simulink model "electromech_dynamics"  (R2020b)
settings: Solver=VariableStepAuto  StartTime=0.0  StopTime=10.0  RelTol=1e-3
values from neighbouring files (symbols this model uses):
  ms22g = 1/g    (= 0.101936799185)    [balrob_params.m]
  Ts = 1e-2    (= 0.01)    [balrob_params.m]
undefined symbols (not defined in the file or in its folder): C12qq_coeff, drv, Fv1, g2_coeff, gbox, M11q, M12q_coeff, M22q, sens, ua2tau1
settings Model: Creator=gioel  LastModifiedBy=gioel

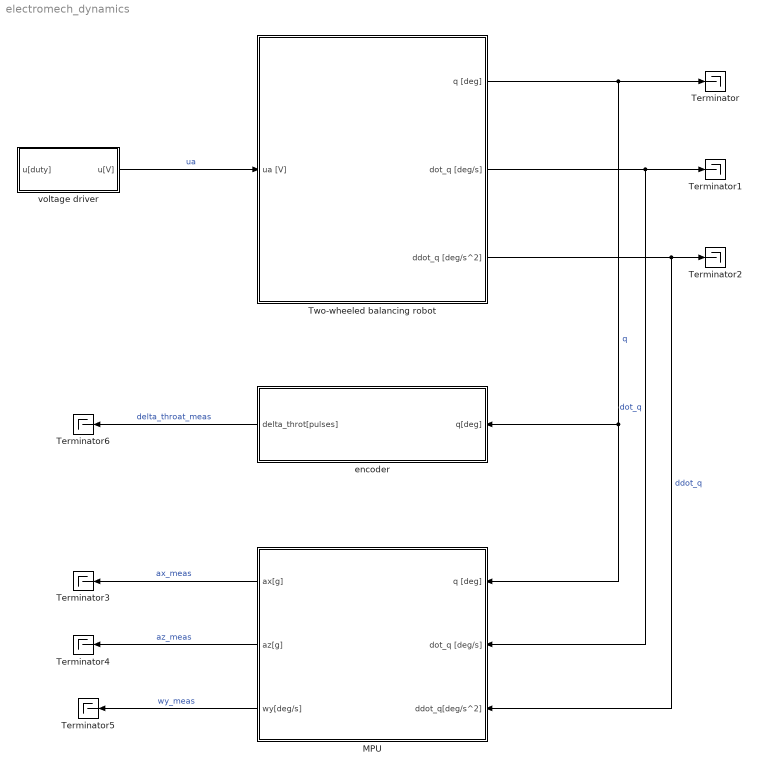
== system electromech_dynamics ==
  MPU : Subsystem
  Terminator{,1..6} (7 alike) : Terminator
  Two-wheeled balancing robot : Subsystem
  encoder : Subsystem
  voltage driver : Subsystem
  wires:
  voltage driver/1(u[V]) -> Two-wheeled balancing robot/1(ua [V])  "ua"
  Two-wheeled balancing robot/1(q [deg]) -> MPU/1(q [deg]), encoder/1(q[deg]), Terminator/1  "q"
  Two-wheeled balancing robot/3(ddot_q [deg/s^2]) -> MPU/3(ddot_q[deg/s^2]), Terminator2/1  "ddot_q"
  Two-wheeled balancing robot/2(dot_q [deg/s]) -> MPU/2(dot_q [deg/s]), Terminator1/1  "dot_q"
  MPU/1(ax[g]) -> Terminator3/1  "ax_meas"
  encoder/1(delta_throt[pulses]) -> Terminator6/1  "delta_throat_meas"
  MPU/2(az[g]) -> Terminator4/1  "az_meas"
  MPU/3(wy[deg/s]) -> Terminator5/1  "wy_meas"

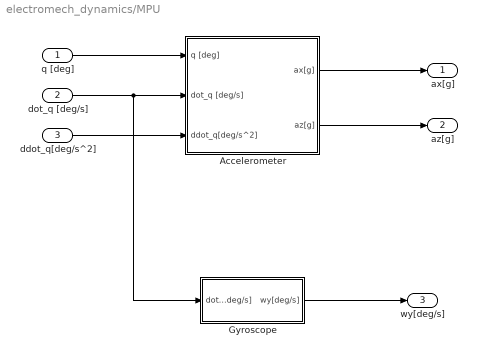
== system electromech_dynamics/MPU ==
  q [deg] : Inport
  dot_q [deg/s] : Inport  Port=2
  ddot_q[deg/s^2] : Inport  Port=3
  Accelerometer : Subsystem
  Gyroscope : Subsystem
  ax[g] : Outport
  az[g] : Outport  Port=2
  wy[deg/s] : Outport  Port=3
  wires:
  q [deg]/1 -> Accelerometer/1(q [deg])
  dot_q [deg/s]/1 -> Gyroscope/1(dot_q [deg/s]), Accelerometer/2(dot_q [deg/s])
  ddot_q[deg/s^2]/1 -> Accelerometer/3(ddot_q[deg/s^2])
  Gyroscope/1(wy[deg/s]) -> wy[deg/s]/1
  Accelerometer/1(ax[g]) -> ax[g]/1
  Accelerometer/2(az[g]) -> az[g]/1

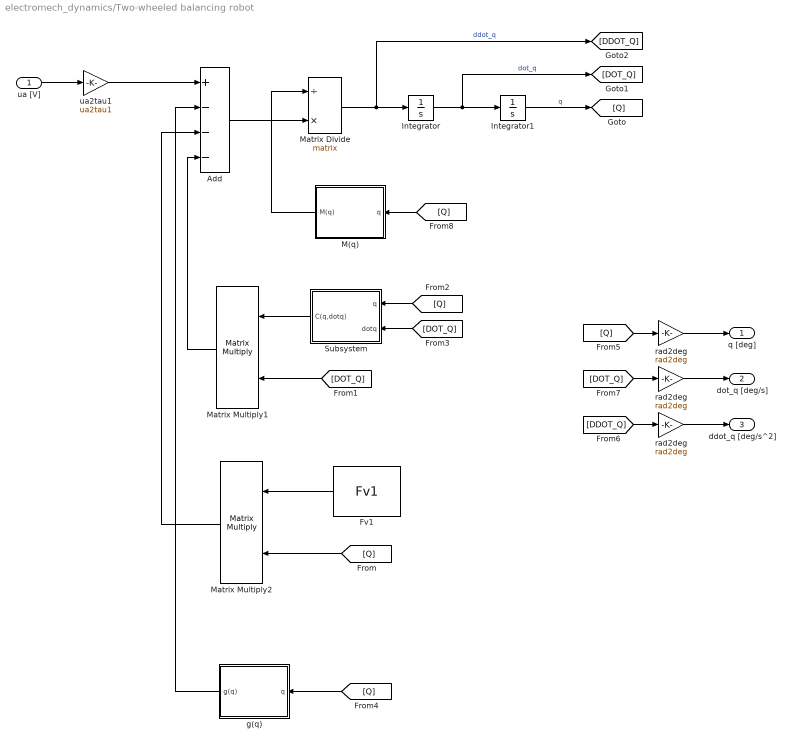
== system electromech_dynamics/Two-wheeled balancing robot ==
  ua [V] : Inport
  Add : Sum  Inputs=+---
  Fv1 : Constant  Value=Fv1
  Integrator : Integrator
  Integrator1 : Integrator
  M(q) : Subsystem
  Matrix Divide : Product  Inputs=/*  Multiplication=Matrix(*)
  Matrix Multiply1 : Product  Multiplication=Matrix(*)
  Matrix Multiply2 : Product  Multiplication=Matrix(*)
  Subsystem : Subsystem
  g(q) : Subsystem
  rad2deg : Gain  Gain=rad2deg
  "rad2deg " : Gain  Gain=rad2deg
  "rad2deg  " : Gain  Gain=rad2deg
  ua2tau1 : Gain  Gain=ua2tau1
  q [deg] : Outport
  dot_q [deg/s] : Outport  Port=2
  ddot_q [deg/s^2] : Outport  Port=3
  wires:
  [DOT_Q] -> "rad2deg  "/1
  [DDOT_Q] -> "rad2deg "/1
  [Q] -> rad2deg/1
  "rad2deg  "/1 -> dot_q [deg/s]/1
  rad2deg/1 -> q [deg]/1
  "rad2deg "/1 -> ddot_q [deg/s^2]/1
  Matrix Divide/1 -> [DDOT_Q], Integrator/1  "ddot_q"
  Add/1 -> Matrix Divide/2
  [Q] -> M(q)/1(q)
  Integrator1/1 -> [Q]  "q"
  [Q] -> Subsystem/1(q)
  ua2tau1/1 -> Add/1
  Subsystem/1(C(q,dotq)) -> Matrix Multiply1/1
  [Q] -> g(q)/1(q)
  Matrix Multiply1/1 -> Add/4
  Integrator/1 -> [DOT_Q], Integrator1/1  "dot_q"
  g(q)/1(g(q)) -> Add/2
  [Q] -> Matrix Multiply2/2
  Matrix Multiply2/1 -> Add/3
  M(q)/1(M(q)) -> Matrix Divide/1
  [DOT_Q] -> Matrix Multiply1/2
  Fv1/1 -> Matrix Multiply2/1
  [DOT_Q] -> Subsystem/2(dotq)
  ua [V]/1 -> ua2tau1/1

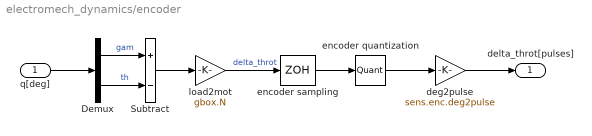
== system electromech_dynamics/encoder ==
  q[deg] : Inport
  Demux : Demux  Outputs=2
  Subtract : Sum  Inputs=+-
  deg2pulse : Gain  Gain=sens.enc.deg2pulse
  encoder quantization : Quantizer  QuantizationInterval=sens.enc.pulse2deg
  encoder sampling : ZeroOrderHold  SampleTime=Ts
  load2mot : Gain  Gain=gbox.N
  delta_throt[pulses] : Outport
  wires:
  q[deg]/1 -> Demux/1
  Demux/1 -> Subtract/1  "gam"
  Demux/2 -> Subtract/2  "th"
  Subtract/1 -> load2mot/1
  load2mot/1 -> encoder sampling/1  "delta_throt"
  encoder sampling/1 -> encoder quantization/1
  encoder quantization/1 -> deg2pulse/1
  deg2pulse/1 -> delta_throt[pulses]/1

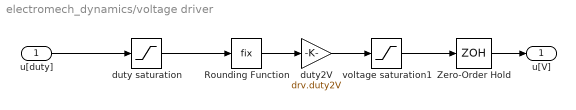
== system electromech_dynamics/voltage driver ==
  u[duty] : Inport
  Rounding Function : Rounding  Operator=fix
  Zero-Order Hold : ZeroOrderHold  SampleTime=Ts
  duty saturation : Saturate  UpperLimit=drv.dutymax  LowerLimit=-drv.dutymax
  duty2V : Gain  Gain=drv.duty2V
  voltage saturation1 : Saturate  UpperLimit=drv.Vbus  LowerLimit=-drv.Vbus
  u[V] : Outport
  wires:
  u[duty]/1 -> duty saturation/1
  duty saturation/1 -> Rounding Function/1
  Rounding Function/1 -> duty2V/1
  duty2V/1 -> voltage saturation1/1
  voltage saturation1/1 -> Zero-Order Hold/1
  Zero-Order Hold/1 -> u[V]/1

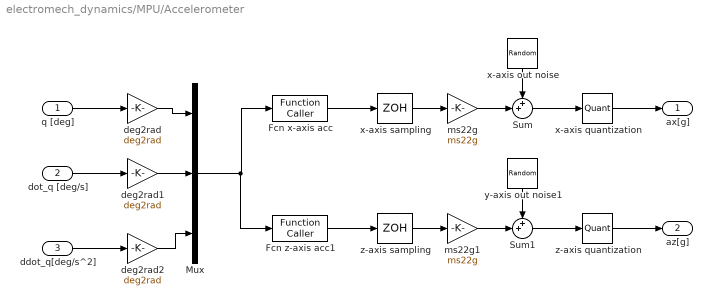
== system electromech_dynamics/MPU/Accelerometer ==
  q [deg] : Inport
  dot_q [deg/s] : Inport  Port=2
  ddot_q[deg/s^2] : Inport  Port=3
  Fcn x-axis acc : FunctionCaller  FunctionPrototype=y = f(u)  InputArgumentSpecifications=<Enter example>  OutputArgumentSpecifications=<Enter example>
  Fcn z-axis acc1 : FunctionCaller  FunctionPrototype=y = f(u)  InputArgumentSpecifications=<Enter example>  OutputArgumentSpecifications=<Enter example>
  Mux : Mux  Inputs=3
  Sum : Sum  Inputs=++|
  Sum1 : Sum  Inputs=++|
  deg2rad : Gain  Gain=deg2rad
  deg2rad1 : Gain  Gain=deg2rad
  deg2rad2 : Gain  Gain=deg2rad
  ms22g : Gain  Gain=ms22g
  ms22g1 : Gain  Gain=ms22g
  x-axis out noise : RandomNumber  Variance=sens.mpu.acc.noisevar  SampleTime=Ts
  x-axis quantization : Quantizer  QuantizationInterval=sens.mpu.acc.LSB2g
  x-axis sampling : ZeroOrderHold  SampleTime=Ts
  y-axis out noise1 : RandomNumber  Variance=sens.mpu.acc.noisevar  SampleTime=Ts
  z-axis quantization : Quantizer  QuantizationInterval=sens.mpu.acc.LSB2g
  z-axis sampling : ZeroOrderHold  SampleTime=Ts
  ax[g] : Outport
  az[g] : Outport  Port=2
  wires:
  ddot_q[deg/s^2]/1 -> deg2rad2/1
  dot_q [deg/s]/1 -> deg2rad1/1
  q [deg]/1 -> deg2rad/1
  deg2rad2/1 -> Mux/3
  deg2rad1/1 -> Mux/2
  deg2rad/1 -> Mux/1
  Mux/1 -> Fcn z-axis acc1/1, Fcn x-axis acc/1
  Fcn z-axis acc1/1 -> z-axis sampling/1
  Fcn x-axis acc/1 -> x-axis sampling/1
  x-axis sampling/1 -> ms22g/1
  z-axis sampling/1 -> ms22g1/1
  x-axis out noise/1 -> Sum/1
  ms22g/1 -> Sum/2
  y-axis out noise1/1 -> Sum1/1
  ms22g1/1 -> Sum1/2
  Sum/1 -> x-axis quantization/1
  Sum1/1 -> z-axis quantization/1
  z-axis quantization/1 -> az[g]/1
  x-axis quantization/1 -> ax[g]/1

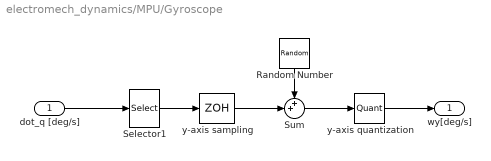
== system electromech_dynamics/MPU/Gyroscope ==
  dot_q [deg/s] : Inport
  Random Number : RandomNumber  Variance=sens.mpu.gyro.noisevar  SampleTime=Ts
  Selector1 : Selector  InputPortWidth=3  IndexOptions=Index vector (dialog)  Indices=[1 3]  OutputSizes=1
  Sum : Sum  Inputs=++|
  y-axis quantization : Quantizer  QuantizationInterval=sens.mpu.gyro.LSB2degs
  y-axis sampling : ZeroOrderHold  SampleTime=Ts
  wy[deg/s] : Outport
  wires:
  dot_q [deg/s]/1 -> Selector1/1
  Selector1/1 -> y-axis sampling/1
  y-axis sampling/1 -> Sum/2
  Random Number/1 -> Sum/1
  Sum/1 -> y-axis quantization/1
  y-axis quantization/1 -> wy[deg/s]/1

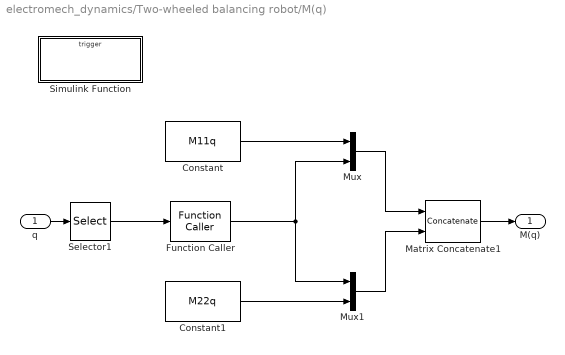
== system electromech_dynamics/Two-wheeled balancing robot/M(q) ==
  q : Inport
  Constant : Constant  Value=M11q
  Constant1 : Constant  Value=M22q
  Function Caller : FunctionCaller  FunctionPrototype=y = M12q(u)  InputArgumentSpecifications=<Enter example>  OutputArgumentSpecifications=<Enter example>
  Matrix Concatenate1 : Concatenate  Mode=Multidimensional array  ConcatenateDimension=2
  Mux : Mux  Inputs=2
  Mux1 : Mux  Inputs=2
  Selector1 : Selector  InputPortWidth=2  IndexOptions=Index vector (dialog)  Indices=2  OutputSizes=1
  Simulink Function : Subsystem  TreatAsAtomicUnit=on
  M(q) : Outport
  wires:
  q/1 -> Selector1/1
  Mux1/1 -> Matrix Concatenate1/2
  Constant1/1 -> Mux1/2
  Mux/1 -> Matrix Concatenate1/1
  Function Caller/1 -> Mux/2, Mux1/1
  Matrix Concatenate1/1 -> M(q)/1
  Selector1/1 -> Function Caller/1
  Constant/1 -> Mux/1

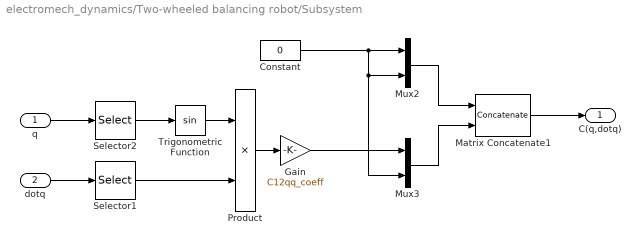
== system electromech_dynamics/Two-wheeled balancing robot/Subsystem ==
  q : Inport
  dotq : Inport  Port=2
  Constant : Constant  Value=0
  Gain : Gain  Gain=C12qq_coeff
  Matrix Concatenate1 : Concatenate  Mode=Multidimensional array  ConcatenateDimension=2
  Mux2 : Mux  Inputs=2
  Mux3 : Mux  Inputs=2
  Product : Product
  Selector1 : Selector  InputPortWidth=2  IndexOptions=Index vector (dialog)  Indices=2  OutputSizes=1
  Selector2 : Selector  InputPortWidth=2  IndexOptions=Index vector (dialog)  Indices=2  OutputSizes=1
  Trigonometric Function : Trigonometry
  C(q,dotq) : Outport
  wires:
  Mux3/1 -> Matrix Concatenate1/2
  Mux2/1 -> Matrix Concatenate1/1
  Constant/1 -> Mux3/2, Mux2/2, Mux2/1
  Matrix Concatenate1/1 -> C(q,dotq)/1
  Gain/1 -> Mux3/1
  q/1 -> Selector2/1
  dotq/1 -> Selector1/1
  Selector1/1 -> Product/2
  Product/1 -> Gain/1
  Trigonometric Function/1 -> Product/1
  Selector2/1 -> Trigonometric Function/1

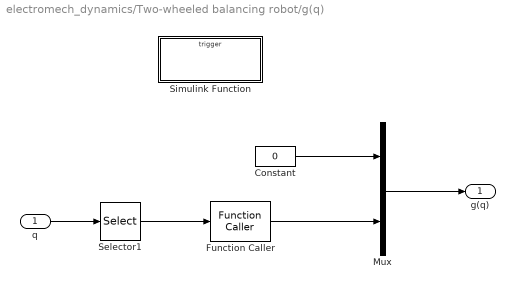
== system electromech_dynamics/Two-wheeled balancing robot/g(q) ==
  q : Inport
  Constant : Constant  Value=0
  Function Caller : FunctionCaller  FunctionPrototype=y = g2(u)  InputArgumentSpecifications=<Enter example>  OutputArgumentSpecifications=<Enter example>
  Mux : Mux  Inputs=2
  Selector1 : Selector  InputPortWidth=2  IndexOptions=Index vector (dialog)  Indices=2  OutputSizes=1
  Simulink Function : Subsystem  TreatAsAtomicUnit=on
  g(q) : Outport
  wires:
  q/1 -> Selector1/1
  Selector1/1 -> Function Caller/1
  Constant/1 -> Mux/1
  Function Caller/1 -> Mux/2
  Mux/1 -> g(q)/1

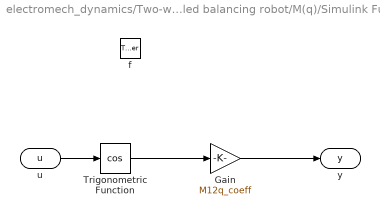
== system electromech_dynamics/Two-wheeled balancing robot/M(q)/Simulink Function ==
  f : TriggerPort  TriggerType=function-call  IsSimulinkFunction=on  FunctionName=M12q  FunctionVisibility=scoped  VariantControl=(inherit)
  Gain : Gain  Gain=M12q_coeff
  Trigonometric Function : Trigonometry  Operator=cos
  u : ArgIn  DisableCoverage=on  ArgumentName=u
  y : ArgOut  DisableCoverage=on  ArgumentName=y
  wires:
  u/1 -> Trigonometric Function/1
  Trigonometric Function/1 -> Gain/1
  Gain/1 -> y/1

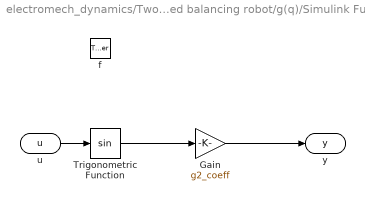
== system electromech_dynamics/Two-wheeled balancing robot/g(q)/Simulink Function ==
  f : TriggerPort  TriggerType=function-call  IsSimulinkFunction=on  FunctionName=g2  FunctionVisibility=scoped  VariantControl=(inherit)
  Gain : Gain  Gain=g2_coeff
  Trigonometric Function : Trigonometry
  u : ArgIn  DisableCoverage=on  ArgumentName=u
  y : ArgOut  DisableCoverage=on  ArgumentName=y
  wires:
  u/1 -> Trigonometric Function/1
  Trigonometric Function/1 -> Gain/1
  Gain/1 -> y/1
